simulink model "s0310_main"  (R2019b)
settings: Solver=FixedStepAuto  StartTime=0.0  StopTime=20  FixedStep=dt  RelTol=1e-3
settings Model: Creator=paolo  LastModifiedBy=francescoceresetti
settings DebuggingCC: SFMachineParentedDataDiag=error  ArithmeticOperatorsInVariantConditions=warning
settings SFSimCC: CustomCodeUndefinedFunction=UseInterfaceOnly
settings CodeAppCC: StateflowObjectComments=on

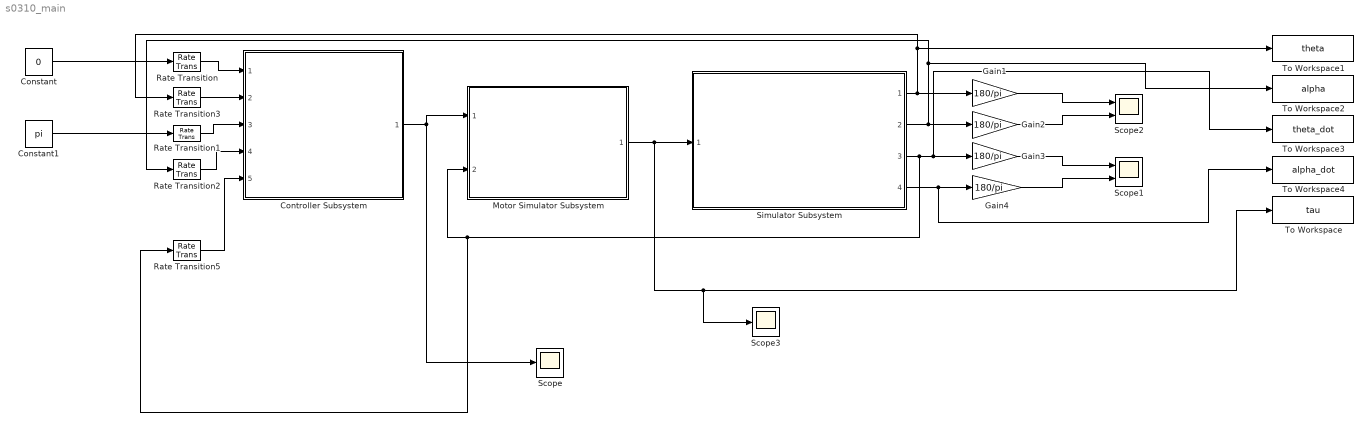
== system s0310_main ==
  Constant : Constant  Value=0
  Constant1 : Constant  Value=pi
  Controller Subsystem : Subsystem  ReferencedSubsystem=s0315_alpha_controller_PP_int  p1=-5  p2=-100  p3=-20
  Gain{1..4} (4 alike) : Gain  Gain=180/pi
  Motor Simulator Subsystem : Subsystem  ReferencedSubsystem=s0303_motor_simulator  omega_0=0  i_0=0
  Rate Transition{,1..3,5} (5 alike) : RateTransition  OutPortSampleTime=dt_control
  Scope : Scope
  Scope1 : Scope  NumInputPorts=2
  Scope2 : Scope  NumInputPorts=2
  Scope3 : Scope
  Simulator Subsystem : Subsystem  ReferencedSubsystem=s0310_simulator  th_0=PARAMS.th_0  al_0=PARAMS.al_0  th_dot_0=PARAMS.th_dot_0  al_dot_0=PARAMS.al_dot_0
  To Workspace : ToWorkspace  VariableName=tau  SampleTime=-1
  To Workspace1 : ToWorkspace  VariableName=theta  SampleTime=-1
  To Workspace2 : ToWorkspace  VariableName=alpha  SampleTime=-1
  To Workspace3 : ToWorkspace  VariableName=theta_dot  SampleTime=-1
  To Workspace4 : ToWorkspace  VariableName=alpha_dot  SampleTime=-1
  wires:
  Simulator Subsystem/1 -> Rate Transition3/1, To Workspace1/1, Gain1/1
  Simulator Subsystem/2 -> Rate Transition2/1, To Workspace2/1, Gain2/1
  Gain1/1 -> Scope2/1
  Gain2/1 -> Scope2/2
  Simulator Subsystem/4 -> To Workspace4/1, Gain4/1
  Gain4/1 -> Scope1/2
  Simulator Subsystem/3 -> Rate Transition5/1, Motor Simulator Subsystem/2, To Workspace3/1, Gain3/1
  Gain3/1 -> Scope1/1
  Motor Simulator Subsystem/1 -> Scope3/1, To Workspace/1, Simulator Subsystem/1
  Constant/1 -> Rate Transition/1
  Constant1/1 -> Rate Transition1/1
  Rate Transition/1 -> Controller Subsystem/1
  Rate Transition3/1 -> Controller Subsystem/2
  Controller Subsystem/1 -> Motor Simulator Subsystem/1, Scope/1
  Rate Transition1/1 -> Controller Subsystem/3
  Rate Transition2/1 -> Controller Subsystem/4
  Rate Transition5/1 -> Controller Subsystem/5
